simulink model "first_system_model"  (R2021b)
settings: Solver=VariableStepAuto  StartTime=0.0  StopTime=10.0  RelTol=1e-3
settings Model: Creator=den  LastModifiedBy=den

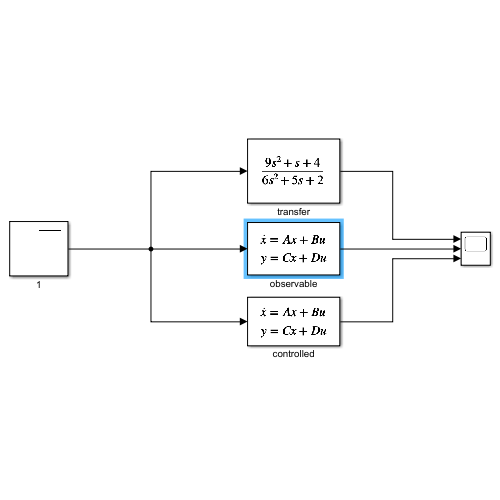
[thumbnail: Simulink's stored preview of the top-level diagram]
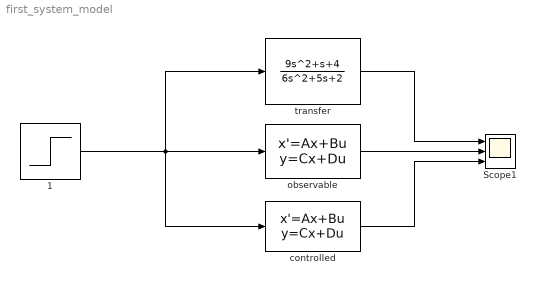
== system first_system_model ==
  1 : Step  Time=0  SampleTime=0
  Scope1 : Scope  NumInputPorts=3
  controlled : StateSpace  A=[0 1; -1/3 -5/6]  B=[0; 1]  C=[1/6 -13/12]  D=3/2  InitialCondition=0
  observable : StateSpace  A=[0 -1/3; 1 -5/6]  B=[1/6; -13/12]  C=[0 1]  D=3/2  InitialCondition=0
  transfer : TransferFcn  Numerator=[9 1 4]  Denominator=[6 5 2]
  wires:
  1/1 -> controlled/1, observable/1, transfer/1
  observable/1 -> Scope1/2
  transfer/1 -> Scope1/1
  controlled/1 -> Scope1/3
